simulink model "ejer4"  (R2015a)
settings: Solver=ode45  StartTime=0.0  StopTime=10.0  RelTol=1e-3
values from neighbouring files (symbols this model uses):
  A = [-1,1;-1,0]    [ejer4.m]
  B = [1;1]    [ejer4.m]
  C = [1,0]    [ejer4.m]
  D = [0]    [ejer4.m]
settings Model: Creator=Sala7  LastModifiedBy=Sala7

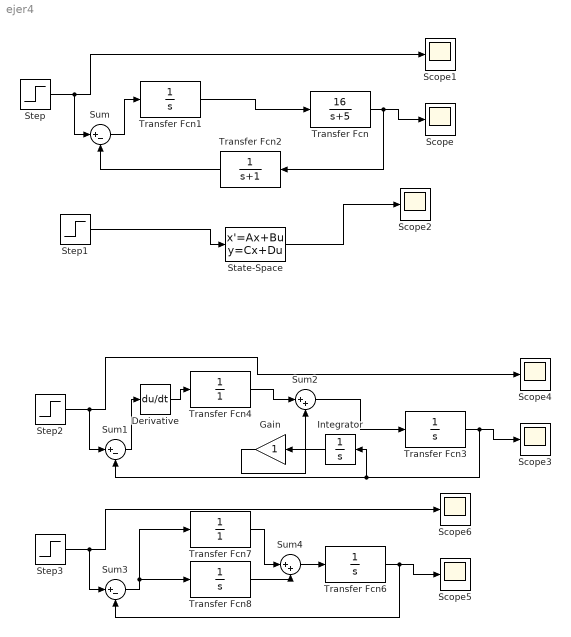
== system ejer4 ==
  Derivative : Derivative
  Gain : Gain
  Integrator : Integrator
  Scope{,1..6} (7 alike) : Scope
      Scope2 settings: SaveName=ScopeData2
      Scope3 settings: SaveName=ScopeData3
      Scope4 settings: SaveName=ScopeData4
      Scope5 settings: SaveName=ScopeData5
      Scope6 settings: SaveName=ScopeData6
  State-Space : StateSpace  A=A  B=B  C=C  D=D  X0=0
  Step{,1..3} (4 alike) : Step  SampleTime=0
  Sum : Sum  Inputs=|+-
  Sum1 : Sum  Inputs=|+-
  Sum2 : Sum  Inputs=|++
  Sum3 : Sum  Inputs=|+-
  Sum4 : Sum  Inputs=|++
  Transfer Fcn : TransferFcn  Numerator=[16]  Denominator=[1 5]
  Transfer Fcn{1,3,6,8} (4 alike) : TransferFcn  Denominator=[1 0]
  Transfer Fcn2 : TransferFcn  Denominator=[1 1]
  Transfer Fcn4 : TransferFcn  Denominator=[1]
  Transfer Fcn7 : TransferFcn  Denominator=[1]
  wires:
  Transfer Fcn/1 -> Transfer Fcn2/1, Scope/1
  Transfer Fcn1/1 -> Transfer Fcn/1
  Step/1 -> Sum/1, Scope1/1
  Sum/1 -> Transfer Fcn1/1
  Transfer Fcn2/1 -> Sum/2
  Step1/1 -> State-Space/1
  State-Space/1 -> Scope2/1
  Step2/1 -> Scope4/1, Sum1/1
  Transfer Fcn3/1 -> Integrator/1, Sum1/2, Scope3/1
  Step3/1 -> Sum3/1, Scope6/1
  Sum3/1 -> Transfer Fcn7/1, Transfer Fcn8/1
  Transfer Fcn6/1 -> Scope5/1, Sum3/2
  Sum4/1 -> Transfer Fcn6/1
  Transfer Fcn7/1 -> Sum4/1
  Transfer Fcn8/1 -> Sum4/2
  Sum1/1 -> Derivative/1
  Derivative/1 -> Transfer Fcn4/1
  Transfer Fcn4/1 -> Sum2/1
  Gain/1 -> Sum2/2
  Sum2/1 -> Transfer Fcn3/1
  Integrator/1 -> Gain/1
